simulink model "Statespace_eqns"  (R2021a)
settings: Solver=VariableStepAuto  StartTime=0.0  StopTime=10.0  RelTol=1e-3
settings Model: Creator=jessilbijou  LastModifiedBy=jessilbijou

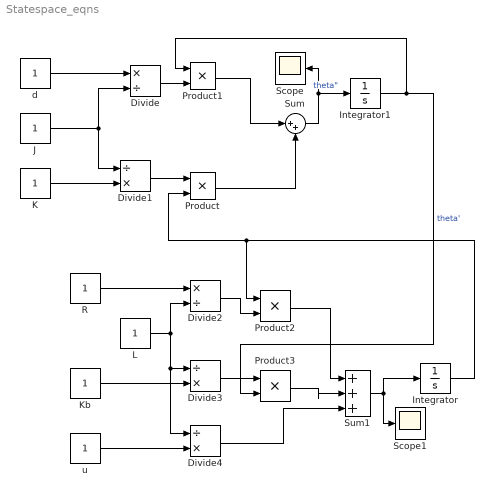
== system Statespace_eqns ==
  Divide : Product  Inputs=*/
  Divide1 : Product  Inputs=/*
  Divide2 : Product  Inputs=*/
  Divide3 : Product  Inputs=/*
  Divide4 : Product  Inputs=/*
  Integrator : Integrator
  Integrator1 : Integrator
  J : Constant
  K : Constant
  Kb : Constant
  L : Constant
  Product{,1..3} (4 alike) : Product
  R : Constant
  Scope : Scope
  Scope1 : Scope
  Sum : Sum  Inputs=|++
  Sum1 : Sum  Inputs=|+++
  d : Constant
  u : Constant
  wires:
  Sum/1 -> Scope/1, Integrator1/1  "theta\""
  Integrator1/1 -> Product1/1, Product3/2  "theta'"
  J/1 -> Divide1/1, Divide/2
  d/1 -> Divide/1
  K/1 -> Divide1/2
  Divide/1 -> Product1/2
  Divide1/1 -> Product/1
  Product/1 -> Sum/2
  Product1/1 -> Sum/1
  R/1 -> Divide2/1
  L/1 -> Divide4/1, Divide3/1, Divide2/2
  Kb/1 -> Divide3/2
  u/1 -> Divide4/2
  Divide3/1 -> Product3/1
  Product2/1 -> Sum1/1
  Product3/1 -> Sum1/2
  Divide4/1 -> Sum1/3
  Sum1/1 -> Integrator/1, Scope1/1
  Integrator/1 -> Product2/1, Product/2
  Divide2/1 -> Product2/2
